simulink model "WhirlyBird_sim"  (R2016a)
settings: Solver=ode45  StartTime=0.0  StopTime=10000  RelTol=1e-3
InitFcn:
  | param
undefined symbols (not defined in the file or in its folder): drawWhirly
libraries: simulink x2
settings Model: Creator=beard  LastModifiedBy=Jacob
settings DataIOCC: LimitDataPoints=on  SaveFormat=Array  SignalLoggingSaveFormat=ModelDataLogs
settings OptimizationCC: ExpressionDepthLimit=2147483647  InitFltsAndDblsToZero=on
settings DebuggingCC: UnderspecifiedInitializationDetection=Classic  MergeDetectMultiDrivingBlocksExec=none  SolverPrmCheckMsg=warning  FcnCallInpInsideContextMsg=UseLocalSettings  StateNameClashWarn=warning
settings HardwareCC: ProdBitPerPointer=32  ProdLargestAtomicFloat=None  ProdIntDivRoundTo=Undefined  ProdEndianess=Unspecified  ProdWordSize=32  ProdHWDeviceType=32-bit Generic
settings ModelReferenceCC: PropagateSignalLabelsOutOfModel=off
settings GRTTargetCC: CombineOutputUpdateFcns=off  GRTInterface=on
settings ConfigComp: CovModelRefEnable=Off

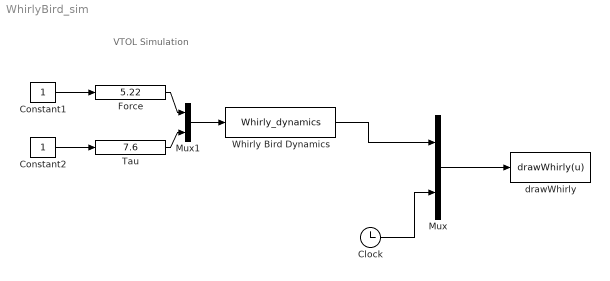
== system WhirlyBird_sim ==
  note: VTOL Simulation
  Clock : Clock
  Constant1 : Constant
  Constant2 : Constant
  Force : simulink/Math Operations/Slider Gain  low=0  gain=5.22  high=12.61
  Mux : Mux  Inputs=2
  Mux1 : Mux  Inputs=2
  Tau : simulink/Math Operations/Slider Gain  low=-0.001  gain=7.6  high=7.6
  Whirly Bird Dynamics : S-Function  FunctionName=Whirly_dynamics  Parameters=P  SFunctionDeploymentMode=off  EnableBusSupport=off
  drawWhirly : MATLABFcn  MATLABFcn=drawWhirly(u)  OutputDimensions=0  SampleTime=0.1
  wires:
  Constant1/1 -> Force/1
  Mux/1 -> drawWhirly/1
  Whirly Bird Dynamics/1 -> Mux/1
  Clock/1 -> Mux/2
  Constant2/1 -> Tau/1
  Mux1/1 -> Whirly Bird Dynamics/1
  Force/1 -> Mux1/1
  Tau/1 -> Mux1/2
